simulink model "lb543_rtlsdr_rx_am_dsb_sc_envelope_demod"  (R2018b)
settings: Solver=VariableStepAuto  StartTime=0.0  StopTime=inf  RelTol=1e-3
undefined symbols (not defined in the file or in its folder): fdesignblkfcn, gcbh
libraries: dspsnks4 x1, dspmlti4 x1, sdrrlib x1
settings Model: SimulationMode=accelerator  Creator=Григорий Фокин  LastModifiedBy=Григорий Фокин
settings SFSimCC: SimUseLocalCustomCode=off
settings RTWCC: RTWUseLocalCustomCode=off
settings CodeAppCC: StateflowObjectComments=on

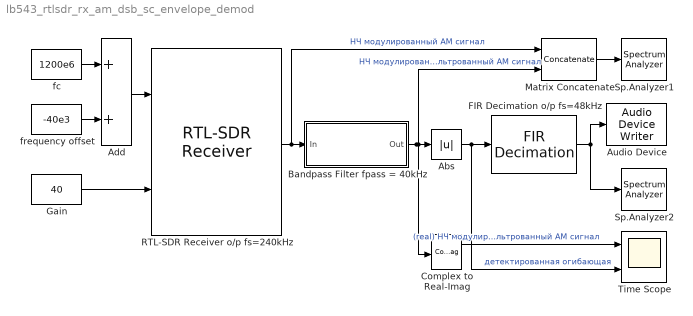
== system lb543_rtlsdr_rx_am_dsb_sc_envelope_demod ==
  Abs : Abs
  Add : Sum
  Audio Device : dspsnks4/Audio Device Writer  Driver=DirectSound  Device=Default  InheritSampleRate=on  SampleRate=44100  BitDepth=16-bit integer  BufferSize=4096  NumBuffers=10  DefaultOutputChannelMapping=on  OutputChannelMapping=1:2  OutputNumUnderrunSamples=off  DriverIdx=1  DeviceWarnFlag=''
  Bandpass Filter fpass = 40kHz : Subsystem  DialogController=fdesignblkfcn  InitFcn=fdesignblkfcn(gcbh, {'InitFcn'});  mask(Bandpass Filter){}
      mask help: Design a bandpass filter
      settings: CopyFcn=fdesignblkfcn(gcbh, {'CopyFcn'});
      mask Help: helpview(mapfilelocation('dsp'), 'dspbandpassfilter');
      mask Display: disp('Bandpass');
  Complex to Real-Imag : ComplexToRealImag
  FIR Decimation o/p fs=48kHz : dspmlti4/FIR Decimation  FilterSource=Dialog parameters  h=firpm(100, [0 15e3 20e3 (240e3/2)]/(240e3/2), [1 1 0 0], [1 1], 20)  D=5  filtStruct=Direct form  FilterObject=FDECIM  InputProcessing=Columns as channels (frame based)  framing=Allow multirate processing  inputOffset=0  outputBufInitCond=0  roundingMode=Floor  overflowMode=off  firstCoeffDataTypeStr=Inherit: Same word length as input  firstCoeffMin=[]  firstCoeffMax=[]  firstCoeffLastDataTypeStr=Inherit: Same word length as input  outputDataTypeStr=Inherit: Same as accumulator  outputMin=[]  outputMax=[]  outputLastDataTypeStr=Inherit: Same as accumulator
  Gain : Constant  Value=40
  Matrix Concatenate : Concatenate  Mode=Multidimensional array  ConcatenateDimension=2
  RTL-SDR Receiver o/p fs=240kHz : sdrrlib/RTL-SDR Receiver  IPAddress=0  CenterFrequencySource=Input port  CenterFrequency=102.5e6  GainSource=Input port  Gain=0  ADCRate=240e3  FrequencyCorrection=47  LostSamplesOutputPort=off  LatencyOutputPort=off  OutputDataType=single  FrameLength=4096  EnableBurstMode=off  NumFramesInBurst=20  sobjType=sdrr.internal.SDRRTLReceiverSL  dataUDPPort=-1  ctrlUDPPort=-1  subDeviceList=nosubdev  sdrBlockType=SDRBlockTypeSLT.SDRRxBlock  requester=UNUSED_BY_SFCN  sdrExecutionMode=SDRExecutionModeSLT.ExecModeHW  BypassUserLogic=off  DecimatorSelect=DDC decimator  SourceSelect=RF data  SineAmplitude=16000  EnableInternalClock=off  BypassIQBalance=off  IFBandwidth=40e6  ADCRateSource=Dialog  IntermediateFrequency=0  DecimationFactorSource=Dialog  DecimationFactor=512  RFFrequencyIsTunable=logical(1)  SampleTime=(4096)/(240e3)  IFBandwidthSource=Dialog  SineFrequency=30000  BypassDCBlockingFilter=off  IntermediateFrequencySource=Dialog  IQBalanceCoefficients=64  SkipAllHardwareResetAndInitialization=off  EnableIQCalibrationTable=on  CacheIQCalibrationTable=off  EnableOffsetTuning=off  EnableRTLAGC=off  EnableTestMode=off  EnableTunerAGC=off  FrequencyCorrectionSource=Dialog  NumMLBuffers=128  NumUSBBuffers=16  RTLCrystalFrequency=28800000  TunerCrystalFrequency=28800000
      settings: SourceProductName=Communications System Toolbox Support Package for RTL-SDR Radio  SourceProductBaseCode=RTLSDR
  Sp.Analyzer1 : SpectrumAnalyzer
  Sp.Analyzer2 : SpectrumAnalyzer
  Time Scope : Scope  NumInputPorts=2
  fc : Constant  Value=1200e6
  frequency offset : Constant  Value=-40e3
  wires:
  Add/1 -> RTL-SDR Receiver o/p fs=240kHz/1
  fc/1 -> Add/1
  frequency offset/1 -> Add/2
  Gain/1 -> RTL-SDR Receiver o/p fs=240kHz/2
  RTL-SDR Receiver o/p fs=240kHz/1 -> Matrix Concatenate/1, Bandpass Filter fpass = 40kHz/1(In)  "НЧ модулированный АМ сигнал"
  Bandpass Filter fpass = 40kHz/1(Out) -> Matrix Concatenate/2, Complex to Real-Imag/1, Abs/1  "НЧ модулированный фильтрованный АМ сигнал"
  Abs/1 -> FIR Decimation o/p fs=48kHz/1, Time Scope/2  "детектированная огибающая"
  FIR Decimation o/p fs=48kHz/1 -> Audio Device/1, Sp.Analyzer2/1
  Matrix Concatenate/1 -> Sp.Analyzer1/1
  Complex to Real-Imag/1 -> Time Scope/1  "(real) НЧ модулированный фильтрованный АМ сигнал"

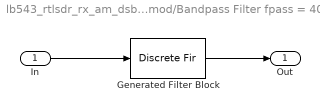
== system lb543_rtlsdr_rx_am_dsb_sc_envelope_demod/Bandpass Filter fpass = 40kHz ==
  In : Inport
  Generated Filter Block : DiscreteFir  Tag=BlockMethodSubSystem  Coefficients=[0.0024383680654391279 -0.0024904844872335181 0.0008296181587990019 0.00075763990941193037 -0.0029743999995476087 -0.0056956755431176575 -0.0028776958737143348 0.0020233577255912068 0.0023310659405153251 -0.00027212204672271616 0.001298980790763055 0.0055550878283859399 0.0037368666021221257 -0.0037077560769040417 -0.00613059502047848 -0.0015673349864665275 -0.00064541981755781273 -0.0058853330339690641 -0.0049754807192339138 0.006058494675769785 0.012134568108140727 0.0046828751969348542 -0.0019634302976165971 0.0030583074049244522 0.0052335956968274488 -0.0081520373462266489 -0.019634505516675459 -0.0095052582270242249 0.0068404420787941383 0.0047887875175383924 -0.0033288481268329327 0.0090952335007955052 0.027639450416940377 0.016192021336710459 -0.015076121972225669 -0.021098373362246688 -0.0027404495183461627 -0.0071585981673002947 -0.034811306082885553 -0.02583264255396283 0.029932696481132618 0.056508405600255517 0.019341104119483532 -0.0029407606412845035 0.039788104942006373 0.047298725684134749 -0.076164128858747751 -0.20720748443321041 -0.12610208390493863 0.14072053470827203 0.29175920861567461 0.14072053470827203 -0.12610208390493863 -0.20720748443321041 -0.076164128858747751 0.047298725684134749 0.039788104942006373 -0.0029407606412845035 0.019341104119483532 0.056508405600255517 0.029932696481132618 -0.02583264255396283 -0.034811306082885553 -0.0071585981673002947 -0.0027404495183461627 -0.021098373362246688 -0.015076121972225669 0.016192021336710459 0.027639450416940377 0.0090952335007955052 -0.0033288481268329327 0.0047887875175383924 0.0068404420787941383 -0.0095052582270242249 -0.019634505516675459 -0.0081520373462266489 0.0052335956968274488 0.0030583074049244522 -0.0019634302976165971 0.0046828751969348542 0.012134568108140727 0.006058494675769785 -0.0049754807192339138 -0.0058853330339690641 -0.00064541981755781273 -0.0015673349864665275 -0.00613059502047848 -0.0037077560769040417 0.0037368666021221257 0.0055550878283859399 0.001298980790763055 -0.00027212204672271616 0.0023310659405153251 0.0020233577255912068 -0.0028776958737143348 -0.0056956755431176575 -0.0029743999995476087 0.00075763990941193037 0.0008296181587990019 -0.0024904844872335181 0.0024383680654391279]  InputProcessing=Columns as channels (frame based)
  Out : Outport
  wires:
  In/1 -> Generated Filter Block/1
  Generated Filter Block/1 -> Out/1
